simulink model "P2PHVDCMMC"  (R2024a)
settings: Solver=FixedStepDiscrete  StartTime=0.0  StopTime=10  RelTol=1e-3
PreLoadFcn:
  | % HVDCMMCInterconnectionParam
StartFcn:
  | tic
StopFcn:
  | toc
values from neighbouring files (symbols this model uses):
  C_PM = 1.758e-3    (= 0.001758)    [P2PHVDCMMCcode.m]
  Cg = 50e-9    (= 5e-08)    [P2PHVDCMMCcode.m]
  Fc = Fnom*3.37    (= 168.5)    [P2PHVDCMMCcode.m]
  Fnom = 50    [P2PHVDCMMCcode.m]
  HRM = 1    [P2PHVDCMMCcode.m]
  Ki_Ireg = 6    [P2PHVDCMMCcode.m]
  Ki_Preg = 1.0    (= 1)    [P2PHVDCMMCcode.m]
  Ki_Qreg = 1.0    (= 1)    [P2PHVDCMMCcode.m]
  Ki_VDCreg = 100    [P2PHVDCMMCcode.m]
  Kp_Ireg = 0.6    [P2PHVDCMMCcode.m]
  Kp_Preg = 0.5/3    (= 0.166666666667)    [P2PHVDCMMCcode.m]
  Kp_Qreg = 0.5/3    (= 0.166666666667)    [P2PHVDCMMCcode.m]
  Kp_VDCreg = 4    [P2PHVDCMMCcode.m]
  L_cable = 15e-3    (= 0.015)    [P2PHVDCMMCcode.m]
  Larm = Larm_pu*(Zb_ac/(2*pi*Fnom))    [P2PHVDCMMCcode.m]
  Larm_pu = 0.15    [P2PHVDCMMCcode.m]
  Lff = Larm_pu/2    (= 0.075)    [P2PHVDCMMCcode.m]
  Limits_Ireg = [ 2.0  -2.0]    [P2PHVDCMMCcode.m]
  Limits_Preg = [ 1.2, 0.8 ]    [P2PHVDCMMCcode.m]
  Limits_Qreg = [ 0.25, -0.25 ]    [P2PHVDCMMCcode.m]
  Limits_VDCreg = [ 2.0  -2.0]    [P2PHVDCMMCcode.m]
  Lxfo = 0.12    [P2PHVDCMMCcode.m]
  N = 6    [P2PHVDCMMCcode.m]
  Nb_PM = 36    [P2PHVDCMMCcode.m]
  Pnom = 1000e6    (= 1000000000)    [P2PHVDCMMCcode.m]
  R_cable = 0.5    [P2PHVDCMMCcode.m]
  R_startup = 400    [P2PHVDCMMCcode.m]
  Rarm = Rarm_pu*Zb_ac    [P2PHVDCMMCcode.m]
  Rff = Rarm_pu/2    (= 0.00075)    [P2PHVDCMMCcode.m]
  Rg = 100    [P2PHVDCMMCcode.m]
  Rxfo = 0.003    [P2PHVDCMMCcode.m]
  Slope_Qref = 0.5    [P2PHVDCMMCcode.m]
  Slope_Vdc_ref = Vnom_dc/5    (= 128000)    [P2PHVDCMMCcode.m]
  Tfault = 9999    [P2PHVDCMMCcode.m]
  Ts = Ts_Control    (= 4e-05)    [P2PHVDCMMCcode.m]
  Ts_Control = 40e-6    (= 4e-05)    [P2PHVDCMMCcode.m]
  Ts_dqn = 2e-5    (= 2e-05)    [P2PHVDCMMCcode.m]
  Ts_Power = 20e-6    (= 2e-05)    [P2PHVDCMMCcode.m]
  Vnom_dc = 640e3    (= 640000)    [P2PHVDCMMCcode.m]
  Vnom_prim = 400e3    (= 400000)    [P2PHVDCMMCcode.m]
  Vnom_sec = 333e3    (= 333000)    [P2PHVDCMMCcode.m]
  Ws = 2*pi*50    (= 314.159265359)    [P2PHVDCMMCcode.m]
undefined symbols (not defined in the file or in its folder): DiscIntNeverNeededParam, Discrete, DQN_Lib, gcbh, Int_DQNc_Mat, Mult_DQNc_Mat, Pcc, S, sps, sps_rtmsupport, spsMeanValueVariableFrequencyModel, spsPLL3phModel, SY3
libraries: simulink x38, spsControlledVoltageSourceLib x30, spsVoltageMeasurementLib x21, spsIdealSwitchLib x21, powerlib_extras x12, spsSecondOrderFilterLib x12, spsCurrentMeasurementLib x12, spsdq0toabcLib x9, spsMeanLib x8, spsMeanVariableFrequencyLib x8, spsabctodq0Lib x8, spsThreePhaseSeriesRLCBranchLib x7
(part 6 of 13)

== system P2PHVDCMMC/MMC AVG_Rec/Circulating current suppression/PI regulator with anti-windup D ==
  note: Anti-windup mechanism: Method of conditionnal integration
      |
      | The integration is suspended if saturation occurs and the
      | control error is of the same sign as the control signal.
      |
      | [1] L.Rundqwist, "Anti-Reset Windup for PID Controllers," Ph.D. Thesis TRFT-1033,
      | Departement of Automatic Control, Lund Institute of Technology, Lund, Sweeden, 1991.
  Error : Inport  SampleTime=Ts
  Compare To Zero : simulink/Logic and Bit Operations/Compare To Zero  relop=>  OutDataTypeStr=uint8  ZeroCross=off
  Compare To Zero1 : simulink/Logic and Bit Operations/Compare To Zero  relop=<  OutDataTypeStr=uint8  ZeroCross=off
  Constant : Constant  Value=0
  Constant1 : Constant  Value=UpperLimit
  Constant3 : Constant  Value=LowerLimit
  Discrete-Time Integrator : DiscreteIntegrator  IntegratorMethod=Integration: Trapezoidal  InitialCondition=Init  SampleTime=Ts  LimitOutput=on  UpperSaturationLimit=UpperLimit  LowerSaturationLimit=LowerLimit  ShowStatePort=on  ICPrevOutput=DiscIntNeverNeededParam  ICPrevScaledInput=DiscIntNeverNeededParam
  Kp4 : Gain  Gain=Kp  SaturateOnIntegerOverflow=on  SampleTime=Ts  OutDataTypeStr=Inherit: Same as input  ParamDataTypeStr=Inherit: Same as input
  Kp5 : Gain  Gain=Ki  SaturateOnIntegerOverflow=on  SampleTime=Ts  OutDataTypeStr=Inherit: Same as input  ParamDataTypeStr=Inherit: Same as input
  Logical Operator : Logic  AllPortsSameDT=off  OutDataTypeStr=boolean
  Logical Operator1 : Logic  AllPortsSameDT=off  OutDataTypeStr=boolean
  Logical Operator2 : Logic  Operator=OR  AllPortsSameDT=off  OutDataTypeStr=boolean
  Relational Operator : RelationalOperator  OutDataTypeStr=boolean  InputSameDT=off
  Relational Operator1 : RelationalOperator  Operator=<=  OutDataTypeStr=boolean  InputSameDT=off
  Saturation2 : Saturate  UpperLimit=UpperLimit  LowerLimit=LowerLimit  SampleTime=Ts
  Sum1 : Sum  InputSameDT=on  SaturateOnIntegerOverflow=on  SampleTime=Ts  OutDataTypeStr=Inherit: Same as first input
  Sum6 : Sum  InputSameDT=on  SaturateOnIntegerOverflow=on  SampleTime=Ts  OutDataTypeStr=Inherit: Same as first input
  Switch : Switch  Criteria=u2 > Threshold  SaturateOnIntegerOverflow=off  InputSameDT=off
  Zero-Order Hold : ZeroOrderHold  SampleTime=Ts
  Out : Outport  SampleTime=Ts  InitialOutput=0
  wires:
  Constant/1 -> Switch/1
  Zero-Order Hold/1 -> Sum1/2, Sum6/1
  Discrete-Time Integrator/State -> Sum1/1
  Sum1/1 -> Relational Operator1/1, Relational Operator/1
  Logical Operator2/1 -> Switch/2
  Relational Operator/1 -> Logical Operator/1  "UpperLimit_is_Reached"
  Relational Operator1/1 -> Logical Operator1/1  "LowerLimit_Is_Reached"
  Constant1/1 -> Relational Operator/2
  Constant3/1 -> Relational Operator1/2
  Compare To Zero/1 -> Logical Operator/2  "Error_is_positive"
  Logical Operator/1 -> Logical Operator2/1
  Logical Operator1/1 -> Logical Operator2/2
  Compare To Zero1/1 -> Logical Operator1/2  "Error_is_negative"
  Error/1 -> Compare To Zero1/1, Compare To Zero/1, Kp4/1, Kp5/1
  Sum6/1 -> Saturation2/1
  Kp4/1 -> Zero-Order Hold/1
  Discrete-Time Integrator/1 -> Sum6/2
  Saturation2/1 -> Out/1
  Switch/1 -> Discrete-Time Integrator/1
  Kp5/1 -> Switch/3

== system P2PHVDCMMC/MMC AVG_Rec/Circulating current suppression/PI regulator with anti-windup D1 ==
  note: Anti-windup mechanism: Method of conditionnal integration
      |
      | The integration is suspended if saturation occurs and the
      | control error is of the same sign as the control signal.
      |
      | [1] L.Rundqwist, "Anti-Reset Windup for PID Controllers," Ph.D. Thesis TRFT-1033,
      | Departement of Automatic Control, Lund Institute of Technology, Lund, Sweeden, 1991.
  Error : Inport  SampleTime=Ts
  Compare To Zero : simulink/Logic and Bit Operations/Compare To Zero  relop=>  OutDataTypeStr=uint8  ZeroCross=off
  Compare To Zero1 : simulink/Logic and Bit Operations/Compare To Zero  relop=<  OutDataTypeStr=uint8  ZeroCross=off
  Constant : Constant  Value=0
  Constant1 : Constant  Value=UpperLimit
  Constant3 : Constant  Value=LowerLimit
  Discrete-Time Integrator : DiscreteIntegrator  IntegratorMethod=Integration: Trapezoidal  InitialCondition=Init  SampleTime=Ts  LimitOutput=on  UpperSaturationLimit=UpperLimit  LowerSaturationLimit=LowerLimit  ShowStatePort=on  ICPrevOutput=DiscIntNeverNeededParam  ICPrevScaledInput=DiscIntNeverNeededParam
  Kp4 : Gain  Gain=Kp  SaturateOnIntegerOverflow=on  SampleTime=Ts  OutDataTypeStr=Inherit: Same as input  ParamDataTypeStr=Inherit: Same as input
  Kp5 : Gain  Gain=Ki  SaturateOnIntegerOverflow=on  SampleTime=Ts  OutDataTypeStr=Inherit: Same as input  ParamDataTypeStr=Inherit: Same as input
  Logical Operator : Logic  AllPortsSameDT=off  OutDataTypeStr=boolean
  Logical Operator1 : Logic  AllPortsSameDT=off  OutDataTypeStr=boolean
  Logical Operator2 : Logic  Operator=OR  AllPortsSameDT=off  OutDataTypeStr=boolean
  Relational Operator : RelationalOperator  OutDataTypeStr=boolean  InputSameDT=off
  Relational Operator1 : RelationalOperator  Operator=<=  OutDataTypeStr=boolean  InputSameDT=off
  Saturation2 : Saturate  UpperLimit=UpperLimit  LowerLimit=LowerLimit  SampleTime=Ts
  Sum1 : Sum  InputSameDT=on  SaturateOnIntegerOverflow=on  SampleTime=Ts  OutDataTypeStr=Inherit: Same as first input
  Sum6 : Sum  InputSameDT=on  SaturateOnIntegerOverflow=on  SampleTime=Ts  OutDataTypeStr=Inherit: Same as first input
  Switch : Switch  Criteria=u2 > Threshold  SaturateOnIntegerOverflow=off  InputSameDT=off
  Zero-Order Hold : ZeroOrderHold  SampleTime=Ts
  Out : Outport  SampleTime=Ts  InitialOutput=0
  wires:
  Kp5/1 -> Switch/3
  Switch/1 -> Discrete-Time Integrator/1
  Saturation2/1 -> Out/1
  Discrete-Time Integrator/1 -> Sum6/2
  Kp4/1 -> Zero-Order Hold/1
  Sum6/1 -> Saturation2/1
  Error/1 -> Kp5/1, Kp4/1, Compare To Zero/1, Compare To Zero1/1
  Compare To Zero1/1 -> Logical Operator1/2  "Error_is_negative"
  Logical Operator1/1 -> Logical Operator2/2
  Logical Operator/1 -> Logical Operator2/1
  Compare To Zero/1 -> Logical Operator/2  "Error_is_positive"
  Constant3/1 -> Relational Operator1/2
  Constant1/1 -> Relational Operator/2
  Relational Operator1/1 -> Logical Operator1/1  "LowerLimit_Is_Reached"
  Relational Operator/1 -> Logical Operator/1  "UpperLimit_is_Reached"
  Logical Operator2/1 -> Switch/2
  Sum1/1 -> Relational Operator/1, Relational Operator1/1
  Discrete-Time Integrator/State -> Sum1/1
  Zero-Order Hold/1 -> Sum6/1, Sum1/2
  Constant/1 -> Switch/1

== system P2PHVDCMMC/MMC AVG_Rec/Subsystem1/Circulating current suppression1 ==
  I_arm : Inport
  wt : Inport  Port=2
  Complex to Real-Imag2 : ComplexToRealImag
  Constant1 : Constant  Value=0
  Constant2 : Constant  Value=0
  Constant4 : Constant  Value=0
  Demux : Demux  Outputs=2
  Gain : Gain  Gain=0*Larm_pu
  Gain1 : Gain  Gain=0*Larm_pu
  Gain2 : Gain  Gain=-2
  I->pu1 : Gain  Gain=0.5  SaturateOnIntegerOverflow=on  OutDataTypeStr=Inherit: Same as input  ParamDataTypeStr=Inherit: Same as input
  I->pu4 : Gain  Gain=sqrt(3)*Vnom_prim/sqrt(2)/Pnom  SaturateOnIntegerOverflow=on  OutDataTypeStr=Inherit: Same as input  ParamDataTypeStr=Inherit: Same as input
  Mux1 : Mux  Inputs=3
  Mux2 : Mux  Inputs=2
  PI regulator with anti-windup D : Subsystem  DialogController=POWERSYS.PowerSysDialog  mask(Discrete PI Controller){Kp=1, Ki=5, Par_Limits=Limits_Ireg, Init=0, Ts=Ts}
      mask prompts: Kp "Proportional gain (Kp):"; Ki "Integral gain (Ki):"; Par_Limits "Output limits: [ Upper   Lower ]"; Init "Output initial value:"; Ts "Sample time:"
      mask help: This block implements a discrete PI controller.
      mask init:
      | UpperLimit=Par_Limits(1);
      | LowerLimit=Par_Limits(2);
      | power_initmask();
      mask Help: This block is part of a subset of blocks in the Extras library that does not have documentation associated with it, other than the block mask description.
      mask Display: disp('PI');
  PI regulator with anti-windup D1 : Subsystem  DialogController=POWERSYS.PowerSysDialog  mask(Discrete PI Controller){Kp=1, Ki=5, Par_Limits=Limits_Ireg, Init=0, Ts=Ts}
      mask prompts: Kp "Proportional gain (Kp):"; Ki "Integral gain (Ki):"; Par_Limits "Output limits: [ Upper   Lower ]"; Init "Output initial value:"; Ts "Sample time:"
      mask help: This block implements a discrete PI controller.
      mask init:
      | UpperLimit=Par_Limits(1);
      | LowerLimit=Par_Limits(2);
      | power_initmask();
      mask Help: This block is part of a subset of blocks in the Extras library that does not have documentation associated with it, other than the block mask description.
      mask Display: disp('PI');
  Rate Transition1 : RateTransition  OutPortSampleTime=Ts_Control
  Saturation1 : Saturate  UpperLimit=2  LowerLimit=-2
  Scope1 : Scope
  Selector1 : Selector  NumberOfDimensions=2  InputPortWidth=3  IndexOptions=Index vector (dialog),Index vector (dialog)  Indices=2,3  OutputSizes=1,1
  Sum1 : Sum  Inputs=-+|
  Sum78 : Sum  Inputs=|++
  Sum83 : Sum  Inputs=-+|
  Sum85 : Sum  Inputs=|+-
  dq0 to abc : spsdq0toabcLib/dq0 to abc  Alignment=90 degrees behind phase A axis
  V_diffi : Outport  VectorParamsAs1DForOutWhenUnconnected=off
  wires:
  I_arm/1 -> Selector1/1
  Gain2/1 -> dq0 to abc/2
  wt/1 -> Gain2/1
  Demux/1 -> Gain/1, Sum85/2
  Gain1/1 -> Sum78/2
  Demux/2 -> Gain1/1, Sum83/1
  dq0 to abc/1 -> Saturation1/1
  Constant1/1 -> Sum83/2
  Sum83/1 -> PI regulator with anti-windup D1/1(Error)
  Sum85/1 -> PI regulator with anti-windup D/1(Error)
  Sum78/1 -> Mux1/1
  Gain/1 -> Sum1/1
  Mux1/1 -> dq0 to abc/1
  PI regulator with anti-windup D/1(Out) -> Sum78/1
  PI regulator with anti-windup D1/1(Out) -> Sum1/2
  Sum1/1 -> Mux1/2
  Constant4/1 -> Mux1/3
  Constant2/1 -> Sum85/1
  Saturation1/1 -> V_diffi/1
  Selector1/1 -> Complex to Real-Imag2/1
  Mux2/1 -> Rate Transition1/1
  Complex to Real-Imag2/2 -> Mux2/2
  Complex to Real-Imag2/1 -> Mux2/1
  Rate Transition1/1 -> I->pu1/1
  I->pu1/1 -> I->pu4/1
  I->pu4/1 -> Demux/1, Scope1/1

== system P2PHVDCMMC/MMC AVG_Rec/Subsystem1/Subsystem ==
  g : Inport
  CVS{1..6} (6 alike) : spsControlledVoltageSourceLib/Controlled Voltage Source  Initialize=off  Source_Type=AC  Amplitude=0  Phase=0  Frequency=0  Measurements=None
  Constant2 : Constant  Value=Vnom_dc/2  SampleTime=Ts_Power
  Ground1 : spsGroundLib/Ground  LConnTagsString=a
  Subsystem : Subsystem
      settings: PortSchema="{\"entries\":[{\"content\":{\"sides\":[{\"content\":{\"connectorIds\":[\"In1\"]},\"type\":\"ConnectorPlacement.EquallySpacedRectSide\",\"uuid\":\"a5cee0a7-b338-4dc7-83bc-48872831f323\"},{\"content\":{\"side\":\"RIGHT\"},\"type\":\"ConnectorPlacement.EquallySpacedRectSide\",\"uuid\":\"ca317b42-2c00-457f-a5f3-7770b49527a9\"},{\"content\":{\"connectorIds\":[\"LConn1\",\"LConn2\",\"LConn3\"],\"side\":\"TOP\"},\"type\":\"ConnectorPlacement.EquallySpacedRectSide\",\"uuid\":\"77de2851-5038-4e86-9464-a1f28ff8b83a\"},{\"content\":{\"connectorIds\":[\"RConn1\",\"RConn2\",\"RConn3\"],\"side\":\"BOTTOM\"},\"type\":\"ConnectorPlacement.EquallySpacedRectSide\",\"uuid\":\"3c356faa-cb69-49bf-bf76-45ac18baf20f\"}]},\"type\":\"ConnectorPlacement.EquallySpacedConnector\",\"uuid\":\"03d4a433-e9ae-4343-977e-c6031a8cb266\"}],\"packageUris\":[\"http://schema.mathworks.com/mf0/Connector/R2020b\"],\"version\":\"1.0\"}"
  Subsystem1 : Subsystem
      settings: PortSchema="{\"entries\":[{\"content\":{\"sides\":[{\"content\":{\"connectorIds\":[\"In1\"]},\"type\":\"ConnectorPlacement.EquallySpacedRectSide\",\"uuid\":\"a5cee0a7-b338-4dc7-83bc-48872831f323\"},{\"content\":{\"side\":\"RIGHT\"},\"type\":\"ConnectorPlacement.EquallySpacedRectSide\",\"uuid\":\"ca317b42-2c00-457f-a5f3-7770b49527a9\"},{\"content\":{\"connectorIds\":[\"LConn1\",\"LConn2\",\"LConn3\"],\"side\":\"TOP\"},\"type\":\"ConnectorPlacement.EquallySpacedRectSide\",\"uuid\":\"77de2851-5038-4e86-9464-a1f28ff8b83a\"},{\"content\":{\"connectorIds\":[\"RConn1\",\"RConn2\",\"RConn3\"],\"side\":\"BOTTOM\"},\"type\":\"ConnectorPlacement.EquallySpacedRectSide\",\"uuid\":\"3c356faa-cb69-49bf-bf76-45ac18baf20f\"}]},\"type\":\"ConnectorPlacement.EquallySpacedConnector\",\"uuid\":\"03d4a433-e9ae-4343-977e-c6031a8cb266\"}],\"packageUris\":[\"http://schema.mathworks.com/mf0/Connector/R2020b\"],\"version\":\"1.0\"}"
  Voltage Measurement1 : spsVoltageMeasurementLib/Voltage Measurement  PhasorSimulation=off  OutputType=Complex  PSBequivalent=0
  Voltage Measurement2 : spsVoltageMeasurementLib/Voltage Measurement  PhasorSimulation=off  OutputType=Complex  PSBequivalent=0
  Voltage Measurement3 : spsVoltageMeasurementLib/Voltage Measurement  PhasorSimulation=off  OutputType=Complex  PSBequivalent=0
  + : PMIOPort  Side=Left
  +1 : PMIOPort  Port=2  Side=Left
  +3 : PMIOPort  Port=3  Side=Left
  - : PMIOPort  Port=4  Side=Right
  -1 : PMIOPort  Port=5  Side=Right
  -2 : PMIOPort  Port=6  Side=Right
  tag scope: Vdc12=global, Vdc13=global, Vdc1=global
  wires:
  Voltage Measurement2/1 -> [Vdc1]
  Voltage Measurement1/1 -> [Vdc12]
  Voltage Measurement3/1 -> [Vdc13]
  Constant2/1 -> CVS4/1, CVS5/1, CVS6/1, CVS1/1, CVS2/1, CVS3/1
  g/1 -> Subsystem/1(g), Subsystem1/1(g)
  connections:
  CVS6/RConn1 -- CVS2/LConn1 -- CVS1/LConn1 -- CVS4/RConn1 -- CVS5/RConn1 -- Ground1/LConn1 -- CVS3/LConn1
  Voltage Measurement2/LConn1 -- Subsystem/LConn1 -- +/RConn1
  Voltage Measurement2/LConn2 -- -/RConn1 -- Subsystem1/RConn1
  Voltage Measurement1/LConn2 -- -1/RConn1 -- Subsystem1/RConn2
  Voltage Measurement3/LConn2 -- Subsystem1/RConn3 -- -2/RConn1
  +1/RConn1 -- Subsystem/LConn2 -- Voltage Measurement1/LConn1
  +3/RConn1 -- Subsystem/LConn3 -- Voltage Measurement3/LConn1
  Subsystem/RConn2 -- CVS2/RConn1
  CVS1/RConn1 -- Subsystem/RConn1
  Subsystem/RConn3 -- CVS3/RConn1
  Subsystem1/LConn1 -- CVS4/LConn1
  Subsystem1/LConn2 -- CVS5/LConn1
  Subsystem1/LConn3 -- CVS6/LConn1

== system P2PHVDCMMC/Subsystem4/ACinv/Circulating current suppression2 ==
  I_arm : Inport
  wt : Inport  Port=2
  Complex to Real-Imag2 : ComplexToRealImag
  Constant1 : Constant  Value=0
  Constant2 : Constant  Value=0
  Constant4 : Constant  Value=0
  Demux : Demux  Outputs=2
  Demux4 : Demux  Outputs=2
  Gain : Gain  Gain=0*Larm_pu
  Gain1 : Gain  Gain=0*Larm_pu
  Gain2 : Gain  Gain=-2
  Gain4 : Gain  Gain=[ [zeros(1,N+4)] ; [0, 0,1 ,zeros(1,N+1)];[zeros(1,N+4)]]
  I->pu1 : Gain  Gain=0.5  SaturateOnIntegerOverflow=on  OutDataTypeStr=Inherit: Same as input  ParamDataTypeStr=Inherit: Same as input
  I->pu4 : Gain  Gain=sqrt(3)*Vnom_prim/sqrt(2)/Pnom  SaturateOnIntegerOverflow=on  OutDataTypeStr=Inherit: Same as input  ParamDataTypeStr=Inherit: Same as input
  Mux1 : Mux  Inputs=3
  Mux2 : Mux  Inputs=2
  Mux3 : Mux  Inputs=2
  PI regulator with anti-windup D : Subsystem  DialogController=POWERSYS.PowerSysDialog  mask(Discrete PI Controller){Kp=1, Ki=5, Par_Limits=Limits_Ireg, Init=0, Ts=Ts}
      mask prompts: Kp "Proportional gain (Kp):"; Ki "Integral gain (Ki):"; Par_Limits "Output limits: [ Upper   Lower ]"; Init "Output initial value:"; Ts "Sample time:"
      mask help: This block implements a discrete PI controller.
      mask init:
      | UpperLimit=Par_Limits(1);
      | LowerLimit=Par_Limits(2);
      | power_initmask();
      mask Help: This block is part of a subset of blocks in the Extras library that does not have documentation associated with it, other than the block mask description.
      mask Display: disp('PI');
  PI regulator with anti-windup D1 : Subsystem  DialogController=POWERSYS.PowerSysDialog  mask(Discrete PI Controller){Kp=1, Ki=5, Par_Limits=Limits_Ireg, Init=0, Ts=Ts}
      mask prompts: Kp "Proportional gain (Kp):"; Ki "Integral gain (Ki):"; Par_Limits "Output limits: [ Upper   Lower ]"; Init "Output initial value:"; Ts "Sample time:"
      mask help: This block implements a discrete PI controller.
      mask init:
      | UpperLimit=Par_Limits(1);
      | LowerLimit=Par_Limits(2);
      | power_initmask();
      mask Help: This block is part of a subset of blocks in the Extras library that does not have documentation associated with it, other than the block mask description.
      mask Display: disp('PI');
  Rate Transition1 : RateTransition  OutPortSampleTime=Ts_Control
  Rate Transition2 : RateTransition  OutPortSampleTime=Ts_Power
  Rate Transition3 : RateTransition  OutPortSampleTime=Ts_Power
  Real-Imag to Complex : RealImagToComplex
  Saturation1 : Saturate  UpperLimit=2  LowerLimit=-2
  Saturation2 : Saturate  UpperLimit=2  LowerLimit=-2
  Scope1 : Scope  Commented=on
  Selector1 : Selector  NumberOfDimensions=2  InputPortWidth=3  IndexOptions=Index vector (dialog),Index vector (dialog)  Indices=2,3  OutputSizes=1,1
  Sum1 : Sum  Inputs=-+|
  Sum78 : Sum  Inputs=|++
  Sum83 : Sum  Inputs=-+|
  Sum85 : Sum  Inputs=|+-
  dq0 to abc : spsdq0toabcLib/dq0 to abc  Alignment=90 degrees behind phase A axis
  V_diffi : Outport  VectorParamsAs1DForOutWhenUnconnected=off
  -2Uref_dq0 : Outport  Port=2
  wires:
  Rate Transition3/1 -> -2Uref_dq0/1
  Rate Transition2/1 -> V_diffi/1
  Mux3/1 -> Saturation2/1
  Real-Imag to Complex/1 -> Gain4/1
  Demux4/2 -> Real-Imag to Complex/2
  Gain4/1 -> Rate Transition3/1
  Demux4/1 -> Real-Imag to Complex/1
  I->pu4/1 -> Scope1/1, Demux/1
  I->pu1/1 -> I->pu4/1
  Rate Transition1/1 -> I->pu1/1
  Complex to Real-Imag2/1 -> Mux2/1
  Complex to Real-Imag2/2 -> Mux2/2
  Mux2/1 -> Rate Transition1/1
  Selector1/1 -> Complex to Real-Imag2/1
  Saturation1/1 -> Rate Transition2/1
  Constant2/1 -> Sum85/1
  Constant4/1 -> Mux1/3
  Sum1/1 -> Mux3/2, Mux1/2
  PI regulator with anti-windup D1/1(Out) -> Sum1/2
  PI regulator with anti-windup D/1(Out) -> Sum78/1
  Mux1/1 -> dq0 to abc/1
  Gain/1 -> Sum1/1
  Sum78/1 -> Mux1/1, Mux3/1
  Sum85/1 -> PI regulator with anti-windup D/1(Error)
  Sum83/1 -> PI regulator with anti-windup D1/1(Error)
  Constant1/1 -> Sum83/2
  dq0 to abc/1 -> Saturation1/1
  Demux/2 -> Sum83/1, Gain1/1
  Gain1/1 -> Sum78/2
  Demux/1 -> Sum85/2, Gain/1
  wt/1 -> Gain2/1
  Gain2/1 -> dq0 to abc/2
  I_arm/1 -> Selector1/1
  Saturation2/1 -> Demux4/1

== system P2PHVDCMMC/Subsystem4/ACrec/Circulating current suppression2 ==
  I_arm : Inport
  wt : Inport  Port=2
  Complex to Real-Imag2 : ComplexToRealImag
  Constant1 : Constant  Value=0
  Constant2 : Constant  Value=0
  Constant4 : Constant  Value=0
  Demux : Demux  Outputs=2
  Demux4 : Demux  Outputs=2
  Gain : Gain  Gain=0*Larm_pu
  Gain1 : Gain  Gain=0*Larm_pu
  Gain2 : Gain  Gain=-2
  Gain3 : Gain  Gain=[ [zeros(1,N+4)] ; [0, 0,1 ,zeros(1,N+1)];[zeros(1,N+4)]]
  I->pu1 : Gain  Gain=0.5  SaturateOnIntegerOverflow=on  OutDataTypeStr=Inherit: Same as input  ParamDataTypeStr=Inherit: Same as input
  I->pu4 : Gain  Gain=sqrt(3)*Vnom_prim/sqrt(2)/Pnom  SaturateOnIntegerOverflow=on  OutDataTypeStr=Inherit: Same as input  ParamDataTypeStr=Inherit: Same as input
  Mux1 : Mux  Inputs=3
  Mux2 : Mux  Inputs=2
  Mux3 : Mux  Inputs=2
  PI regulator with anti-windup D : Subsystem  DialogController=POWERSYS.PowerSysDialog  mask(Discrete PI Controller){Kp=1, Ki=5, Par_Limits=Limits_Ireg, Init=0, Ts=Ts}
      mask prompts: Kp "Proportional gain (Kp):"; Ki "Integral gain (Ki):"; Par_Limits "Output limits: [ Upper   Lower ]"; Init "Output initial value:"; Ts "Sample time:"
      mask help: This block implements a discrete PI controller.
      mask init:
      | UpperLimit=Par_Limits(1);
      | LowerLimit=Par_Limits(2);
      | power_initmask();
      mask Help: This block is part of a subset of blocks in the Extras library that does not have documentation associated with it, other than the block mask description.
      mask Display: disp('PI');
  PI regulator with anti-windup D1 : Subsystem  DialogController=POWERSYS.PowerSysDialog  mask(Discrete PI Controller){Kp=1, Ki=5, Par_Limits=Limits_Ireg, Init=0, Ts=Ts}
      mask prompts: Kp "Proportional gain (Kp):"; Ki "Integral gain (Ki):"; Par_Limits "Output limits: [ Upper   Lower ]"; Init "Output initial value:"; Ts "Sample time:"
      mask help: This block implements a discrete PI controller.
      mask init:
      | UpperLimit=Par_Limits(1);
      | LowerLimit=Par_Limits(2);
      | power_initmask();
      mask Help: This block is part of a subset of blocks in the Extras library that does not have documentation associated with it, other than the block mask description.
      mask Display: disp('PI');
  Rate Transition1 : RateTransition  OutPortSampleTime=Ts_Control
  Rate Transition2 : RateTransition  OutPortSampleTime=Ts_Power
  Rate Transition3 : RateTransition  OutPortSampleTime=Ts_Power
  Real-Imag to Complex : RealImagToComplex
  Saturation1 : Saturate  UpperLimit=2  LowerLimit=-2
  Saturation2 : Saturate  UpperLimit=2  LowerLimit=-2
  Scope1 : Scope  Commented=on
  Selector1 : Selector  NumberOfDimensions=2  InputPortWidth=3  IndexOptions=Index vector (dialog),Index vector (dialog)  Indices=2,3  OutputSizes=1,1
  Sum1 : Sum  Inputs=-+|
  Sum78 : Sum  Inputs=|++
  Sum83 : Sum  Inputs=-+|
  Sum85 : Sum  Inputs=|+-
  dq0 to abc : spsdq0toabcLib/dq0 to abc  Alignment=90 degrees behind phase A axis
  V_diffi : Outport  VectorParamsAs1DForOutWhenUnconnected=off
  -2Uref_dq0 : Outport  Port=2
  wires:
  Saturation2/1 -> Demux4/1
  I_arm/1 -> Selector1/1
  Gain2/1 -> dq0 to abc/2
  wt/1 -> Gain2/1
  Demux/1 -> Gain/1, Sum85/2
  Gain1/1 -> Sum78/2
  Demux/2 -> Gain1/1, Sum83/1
  dq0 to abc/1 -> Saturation1/1
  Constant1/1 -> Sum83/2
  Sum83/1 -> PI regulator with anti-windup D1/1(Error)
  Sum85/1 -> PI regulator with anti-windup D/1(Error)
  Sum78/1 -> Mux3/1, Mux1/1
  Gain/1 -> Sum1/1
  Mux1/1 -> dq0 to abc/1
  PI regulator with anti-windup D/1(Out) -> Sum78/1
  PI regulator with anti-windup D1/1(Out) -> Sum1/2
  Sum1/1 -> Mux1/2, Mux3/2
  Constant4/1 -> Mux1/3
  Constant2/1 -> Sum85/1
  Saturation1/1 -> Rate Transition2/1
  Selector1/1 -> Complex to Real-Imag2/1
  Mux2/1 -> Rate Transition1/1
  Complex to Real-Imag2/2 -> Mux2/2
  Complex to Real-Imag2/1 -> Mux2/1
  Rate Transition1/1 -> I->pu1/1
  I->pu1/1 -> I->pu4/1
  I->pu4/1 -> Demux/1, Scope1/1
  Demux4/1 -> Real-Imag to Complex/1
  Gain3/1 -> Rate Transition3/1
  Demux4/2 -> Real-Imag to Complex/2
  Real-Imag to Complex/1 -> Gain3/1
  Mux3/1 -> Saturation2/1
  Rate Transition2/1 -> V_diffi/1
  Rate Transition3/1 -> -2Uref_dq0/1

== system P2PHVDCMMC/Control _DQn_inv/PLL, Measurements and Transformation1/PLL (3ph)/Model ==
  note: vq
  Vdq : Inport
  Automatic Gain Control : Subsystem  TreatAsAtomicUnit=on
  Constant1 : Constant  Value=sps.AGC  SampleTime=Ts
  Constant4 : Constant  Value=2*pi  SampleTime=Ts
  Discrete : Subsystem  DialogController=POWERSYS.PowerSysDialog  VariantControl=PID_Discrete  mask(Discrete PID Controller){Kp=sps.Kp, Ki=sps.Ki, Kd=sps.Kd, TcD=sps.TcD, Par_Limits=[inf 0], Init=2*pi*sps.Finit, Ts=Ts}
      mask prompts: Kp "Proportional gain (Kp):"; Ki "Integral gain (Ki):"; Kd "Derivative gain (Kd):"; TcD "Time constant for derivative filter (s):"; Par_Limits "Output limits: [ Upper   Lower ]"; Init "Output initial value:"; Ts "Sample time:"
      mask help: This block implements a discrete PID controller.
      mask Display: disp('PID');
  Discrete-Time Integrator : DiscreteIntegrator  ExternalReset=rising  InitialConditionSource=external  InitialCondition=sps.Phase_Init*pi/180  SampleTime=Ts  ShowStatePort=on  ICPrevOutput=DiscIntNeverNeededParam  ICPrevScaledInput=DiscIntNeverNeededParam
  Divide : Product
  Gain10 : Gain  Gain=1/2/pi  SaturateOnIntegerOverflow=on  OutDataTypeStr=Inherit: Same as input  ParamDataTypeStr=Inherit: Same as input
  Initial : InitialCondition  Value=sps.Phase_Init*pi/180
  Rate Limiter : RateLimiter  RisingSlewLimit=sps.MaxRateChangeFreq  FallingSlewLimit=-sps.MaxRateChangeFreq  SampleTimeMode=inherited  InitialCondition=sps.Finit
  Relational Operator : RelationalOperator  Operator=>  OutDataTypeStr=boolean  InputSameDT=off
  Second-Order Filter : spsSecondOrderFilterLib/Second-Order Filter  FilterType=Lowpass  Fo=sps.FilterCutOffFreq  Zeta=0.707  Ts=Ts  Initialize=on  Vac_Init=[0 0 sps.Finit]  Vdc_Init=sps.Finit  PlotResponse=off  FreqRange=[1 500 1]
      settings: LibrarySourceBlock=|
      | sps_lib/Control/Filters/Second-Order
      | Filter
  Selector : Selector  Commented=on  InputPortWidth=3  IndexOptions=Index vector (dialog)  Indices=2  OutputSizes=1
  Selector1 : Selector  InputPortWidth=2  IndexOptions=Index vector (dialog)  Indices=2  OutputSizes=1
  Subtract : Sum  Inputs=+-
  Unit Delay : UnitDelay  InitialCondition=sps.Finit  SampleTime=Ts  HasFrameUpgradeWarning=on
  Variable Frequency Mean value : Subsystem  AncestorBlock=|  DialogController=POWERSYS.PowerSysDialog  LoadFcn=sps_rtmsupport('LoadFcn', gcbh);  StartFcn=sps_rtmsupport('StartFcn', gcbh);  StopFcn=sps_rtmsupport('StopFcn', gcbh);  mask(Mean (Variable Frequency)){Finit=sps.Finit, Fmin=sps.Fmin, Vinit=0, Ts=Ts}
      | sps_lib/Sensors and Measurements/Mean
      | (Variable Frequency)
      mask prompts: Finit "Initial frequency (Hz):"; Fmin "Minimum frequency (Hz):"; Vinit "Initial input (DC component):"; Ts "Sample time:"
      mask help:
      | Compute the mean value of input 2 over a running window of one cycle of frequency signal given by input 1.
      |
      | For the first cycle of initial frequency, the output is held to the value specified in the Initial input (DC component) parameter.
      |
      | The Minimum frequency parameter is used to determine the buffer size of the Variable Time Delay block used under the mask of the block.
      mask init:
      | block=gcb;
      | [WantBlockChoice,Ts,sps] = powericon('MeanVariableFrequencyInit',block,Finit,Fmin,Vinit,Ts);
      | powericon('SetInternalModels','set',block,WantBlockChoice);
      settings: CopyFcn=sps_rtmsupport('CopyFcn', gcbh);  DeleteFcn=sps_rtmsupport('DeleteFcn', gcbh);  UndoDeleteFcn=sps_rtmsupport('UndoDeleteFcn', gcbh);  ModelCloseFcn=sps_rtmsupport('ModelCloseFcn', gcbh);  PreSaveFcn=sps_rtmsupport('PreSaveFcn', gcbh);  PostSaveFcn=sps_rtmsupport('PostSaveFcn', gcbh);  NameChangeFcn=sps_rtmsupport('NameChangeFcn', gcbh);  PreCopyFcn=sps_rtmsupport('PreCopyFcn', gcbh);  OpenFcn=sps_rtmsupport('OpenFcn', gcbh, []);  CloseFcn=sps_rtmsupport('CloseFcn', gcbh);  PreDeleteFcn=sps_rtmsupport('PreDeleteFcn', gcbh);
      settings: LibrarySourceBlock=|
      | sps_lib/Sensors and Measurements/Mean
      | (Variable Frequency)
      mask Help: helpview(psbhelp);
      mask Display:
      | port_label('input',1,'Freq')
      | port_label('input',2,'In')
      | plot(0,0, 1,1)
      | plot([0.8 1], [0.75 0.75])
      | plot([0.85 .95], [0.35 0.65],[0.85 .95], [0.65 0.35])
  abc to dq0 : spsabctodq0Lib/abc to dq0  Commented=on  Alignment=90 degrees behind phase A axis
  Freq : Outport  VectorParamsAs1DForOutWhenUnconnected=off
  wt : Outport  Port=2  VectorParamsAs1DForOutWhenUnconnected=off
  wires:
  Rate Limiter/1 -> Second-Order Filter/1
  Gain10/1 -> Rate Limiter/1
  Vdq/1 -> Automatic Gain Control/2(Vdq), Selector1/1
  Second-Order Filter/1 -> Unit Delay/1
  Unit Delay/1 -> Automatic Gain Control/1(Freq), Variable Frequency Mean value/1(Freq), Freq/1
  Discrete-Time Integrator/1 -> wt/1
  Constant4/1 -> Subtract/2, Relational Operator/2
  abc to dq0/1 -> Selector/1
  Discrete/1(Out) -> Gain10/1, Discrete-Time Integrator/1  "W"
  Variable Frequency Mean value/1(Mean) -> Divide/1
  Automatic Gain Control/1(Gain) -> Divide/2
  Divide/1 -> Discrete/1(Err)
  Constant1/1 -> Automatic Gain Control/Enable
  Relational Operator/1 -> Discrete-Time Integrator/2
  Discrete-Time Integrator/State -> Subtract/1, Relational Operator/1
  Subtract/1 -> Initial/1
  Initial/1 -> Discrete-Time Integrator/3
  Selector1/1 -> Variable Frequency Mean value/2(vq)

== system P2PHVDCMMC/Control _DQn_inv/PLL, Measurements and Transformation1/PLL (3ph)2/Model ==
  note: vq
  Vdq : Inport
  Automatic Gain Control : Subsystem  TreatAsAtomicUnit=on
  Constant1 : Constant  Value=sps.AGC  SampleTime=Ts
  Constant4 : Constant  Value=2*pi  SampleTime=Ts
  Discrete : Subsystem  DialogController=POWERSYS.PowerSysDialog  VariantControl=PID_Discrete  mask(Discrete PID Controller){Kp=sps.Kp, Ki=sps.Ki, Kd=sps.Kd, TcD=sps.TcD, Par_Limits=[inf 0], Init=2*pi*sps.Finit, Ts=Ts}
      mask prompts: Kp "Proportional gain (Kp):"; Ki "Integral gain (Ki):"; Kd "Derivative gain (Kd):"; TcD "Time constant for derivative filter (s):"; Par_Limits "Output limits: [ Upper   Lower ]"; Init "Output initial value:"; Ts "Sample time:"
      mask help: This block implements a discrete PID controller.
      mask Display: disp('PID');
  Discrete-Time Integrator : DiscreteIntegrator  ExternalReset=rising  InitialConditionSource=external  InitialCondition=sps.Phase_Init*pi/180  SampleTime=Ts  ShowStatePort=on  ICPrevOutput=DiscIntNeverNeededParam  ICPrevScaledInput=DiscIntNeverNeededParam
  Divide : Product
  Gain10 : Gain  Gain=1/2/pi  SaturateOnIntegerOverflow=on  OutDataTypeStr=Inherit: Same as input  ParamDataTypeStr=Inherit: Same as input
  Initial : InitialCondition  Value=sps.Phase_Init*pi/180
  MATLAB Function : MATLAB Function  TreatAsAtomicUnit=on
  Mux : Mux  Inputs=2
  Rate Limiter : RateLimiter  RisingSlewLimit=sps.MaxRateChangeFreq  FallingSlewLimit=-sps.MaxRateChangeFreq  SampleTimeMode=inherited  InitialCondition=sps.Finit
  Rate Transition3 : RateTransition  OutPortSampleTime=Ts_Control
  Relational Operator : RelationalOperator  Operator=>  OutDataTypeStr=boolean  InputSameDT=off
  Second-Order Filter : spsSecondOrderFilterLib/Second-Order Filter  FilterType=Lowpass  Fo=sps.FilterCutOffFreq  Zeta=0.707  Ts=Ts  Initialize=on  Vac_Init=[0 0 sps.Finit]  Vdc_Init=sps.Finit  PlotResponse=off  FreqRange=[1 500 1]
      settings: LibrarySourceBlock=|
      | sps_lib/Control/Filters/Second-Order
      | Filter
  Selector1 : Selector  InputPortWidth=2  IndexOptions=Index vector (dialog)  Indices=2  OutputSizes=1
  Subtract : Sum  Inputs=+-
  Sum : Sum  Inputs=|+-
  Unit Delay : UnitDelay  InitialCondition=sps.Finit  SampleTime=Ts  HasFrameUpgradeWarning=on
  Variable Frequency Mean value : Subsystem  AncestorBlock=|  DialogController=POWERSYS.PowerSysDialog  LoadFcn=sps_rtmsupport('LoadFcn', gcbh);  StartFcn=sps_rtmsupport('StartFcn', gcbh);  StopFcn=sps_rtmsupport('StopFcn', gcbh);  mask(Mean (Variable Frequency)){Finit=sps.Finit, Fmin=sps.Fmin, Vinit=0, Ts=Ts}
      | sps_lib/Sensors and Measurements/Mean
      | (Variable Frequency)
      mask prompts: Finit "Initial frequency (Hz):"; Fmin "Minimum frequency (Hz):"; Vinit "Initial input (DC component):"; Ts "Sample time:"
      mask help:
      | Compute the mean value of input 2 over a running window of one cycle of frequency signal given by input 1.
      |
      | For the first cycle of initial frequency, the output is held to the value specified in the Initial input (DC component) parameter.
      |
      | The Minimum frequency parameter is used to determine the buffer size of the Variable Time Delay block used under the mask of the block.
      mask init:
      | block=gcb;
      | [WantBlockChoice,Ts,sps] = powericon('MeanVariableFrequencyInit',block,Finit,Fmin,Vinit,Ts);
      | powericon('SetInternalModels','set',block,WantBlockChoice);
      settings: CopyFcn=sps_rtmsupport('CopyFcn', gcbh);  DeleteFcn=sps_rtmsupport('DeleteFcn', gcbh);  UndoDeleteFcn=sps_rtmsupport('UndoDeleteFcn', gcbh);  ModelCloseFcn=sps_rtmsupport('ModelCloseFcn', gcbh);  PreSaveFcn=sps_rtmsupport('PreSaveFcn', gcbh);  PostSaveFcn=sps_rtmsupport('PostSaveFcn', gcbh);  NameChangeFcn=sps_rtmsupport('NameChangeFcn', gcbh);  PreCopyFcn=sps_rtmsupport('PreCopyFcn', gcbh);  OpenFcn=sps_rtmsupport('OpenFcn', gcbh, []);  CloseFcn=sps_rtmsupport('CloseFcn', gcbh);  PreDeleteFcn=sps_rtmsupport('PreDeleteFcn', gcbh);
      settings: LibrarySourceBlock=|
      | sps_lib/Sensors and Measurements/Mean
      | (Variable Frequency)
      mask Help: helpview(psbhelp);
      mask Display:
      | port_label('input',1,'Freq')
      | port_label('input',2,'In')
      | plot(0,0, 1,1)
      | plot([0.8 1], [0.75 0.75])
      | plot([0.85 .95], [0.35 0.65],[0.85 .95], [0.65 0.35])
  Freq : Outport  VectorParamsAs1DForOutWhenUnconnected=off
  wt : Outport  Port=2  VectorParamsAs1DForOutWhenUnconnected=off
  wires:
  Rate Limiter/1 -> Second-Order Filter/1
  Gain10/1 -> Rate Limiter/1
  Second-Order Filter/1 -> Unit Delay/1
  Unit Delay/1 -> Automatic Gain Control/1(Freq), Variable Frequency Mean value/1(Freq), Freq/1
  Constant4/1 -> Subtract/2, Relational Operator/2
  Discrete/1(Out) -> Gain10/1, Discrete-Time Integrator/1  "W"
  Variable Frequency Mean value/1(Mean) -> Divide/1
  Automatic Gain Control/1(Gain) -> Divide/2
  Divide/1 -> Discrete/1(Err)
  Constant1/1 -> Automatic Gain Control/Enable
  Relational Operator/1 -> Discrete-Time Integrator/2
  Discrete-Time Integrator/State -> Subtract/1, Relational Operator/1
  Subtract/1 -> Initial/1
  Initial/1 -> Discrete-Time Integrator/3
  Selector1/1 -> Variable Frequency Mean value/2(vq)
  Sum/1 -> MATLAB Function/2(wt)
  Discrete-Time Integrator/1 -> Sum/1, wt/1
  MATLAB Function/1(d) -> Mux/1
  MATLAB Function/2(q) -> Mux/2
  Mux/1 -> Automatic Gain Control/2(Vdq), Selector1/1
  Vdq/1 -> MATLAB Function/1(DQ)
  [wt0] -> Rate Transition3/1
  Rate Transition3/1 -> Sum/2

== system P2PHVDCMMC/Control _DQn_rec/PLL, Measurements and Transformation1/PLL (3ph)/Model ==
  note: vq
  Vdq : Inport
  Automatic Gain Control : Subsystem  TreatAsAtomicUnit=on
  Constant1 : Constant  Value=sps.AGC  SampleTime=Ts
  Constant4 : Constant  Value=2*pi  SampleTime=Ts
  Discrete : Subsystem  DialogController=POWERSYS.PowerSysDialog  VariantControl=PID_Discrete  mask(Discrete PID Controller){Kp=sps.Kp, Ki=sps.Ki, Kd=sps.Kd, TcD=sps.TcD, Par_Limits=[inf 0], Init=2*pi*sps.Finit, Ts=Ts}
      mask prompts: Kp "Proportional gain (Kp):"; Ki "Integral gain (Ki):"; Kd "Derivative gain (Kd):"; TcD "Time constant for derivative filter (s):"; Par_Limits "Output limits: [ Upper   Lower ]"; Init "Output initial value:"; Ts "Sample time:"
      mask help: This block implements a discrete PID controller.
      mask Display: disp('PID');
  Discrete-Time Integrator : DiscreteIntegrator  ExternalReset=rising  InitialConditionSource=external  InitialCondition=sps.Phase_Init*pi/180  SampleTime=Ts  ShowStatePort=on  ICPrevOutput=DiscIntNeverNeededParam  ICPrevScaledInput=DiscIntNeverNeededParam
  Divide : Product
  Gain10 : Gain  Gain=1/2/pi  SaturateOnIntegerOverflow=on  OutDataTypeStr=Inherit: Same as input  ParamDataTypeStr=Inherit: Same as input
  Initial : InitialCondition  Value=sps.Phase_Init*pi/180
  Rate Limiter : RateLimiter  RisingSlewLimit=sps.MaxRateChangeFreq  FallingSlewLimit=-sps.MaxRateChangeFreq  SampleTimeMode=inherited  InitialCondition=sps.Finit
  Relational Operator : RelationalOperator  Operator=>  OutDataTypeStr=boolean  InputSameDT=off
  Second-Order Filter : spsSecondOrderFilterLib/Second-Order Filter  FilterType=Lowpass  Fo=sps.FilterCutOffFreq  Zeta=0.707  Ts=Ts  Initialize=on  Vac_Init=[0 0 sps.Finit]  Vdc_Init=sps.Finit  PlotResponse=off  FreqRange=[1 500 1]
      settings: LibrarySourceBlock=|
      | sps_lib/Control/Filters/Second-Order
      | Filter
  Selector : Selector  Commented=on  InputPortWidth=3  IndexOptions=Index vector (dialog)  Indices=2  OutputSizes=1
  Selector1 : Selector  InputPortWidth=2  IndexOptions=Index vector (dialog)  Indices=2  OutputSizes=1
  Subtract : Sum  Inputs=+-
  Unit Delay : UnitDelay  InitialCondition=sps.Finit  SampleTime=Ts  HasFrameUpgradeWarning=on
  Variable Frequency Mean value : Subsystem  AncestorBlock=|  DialogController=POWERSYS.PowerSysDialog  LoadFcn=sps_rtmsupport('LoadFcn', gcbh);  StartFcn=sps_rtmsupport('StartFcn', gcbh);  StopFcn=sps_rtmsupport('StopFcn', gcbh);  mask(Mean (Variable Frequency)){Finit=sps.Finit, Fmin=sps.Fmin, Vinit=0, Ts=Ts}
      | sps_lib/Sensors and Measurements/Mean
      | (Variable Frequency)
      mask prompts: Finit "Initial frequency (Hz):"; Fmin "Minimum frequency (Hz):"; Vinit "Initial input (DC component):"; Ts "Sample time:"
      mask help:
      | Compute the mean value of input 2 over a running window of one cycle of frequency signal given by input 1.
      |
      | For the first cycle of initial frequency, the output is held to the value specified in the Initial input (DC component) parameter.
      |
      | The Minimum frequency parameter is used to determine the buffer size of the Variable Time Delay block used under the mask of the block.
      mask init:
      | block=gcb;
      | [WantBlockChoice,Ts,sps] = powericon('MeanVariableFrequencyInit',block,Finit,Fmin,Vinit,Ts);
      | powericon('SetInternalModels','set',block,WantBlockChoice);
      settings: CopyFcn=sps_rtmsupport('CopyFcn', gcbh);  DeleteFcn=sps_rtmsupport('DeleteFcn', gcbh);  UndoDeleteFcn=sps_rtmsupport('UndoDeleteFcn', gcbh);  ModelCloseFcn=sps_rtmsupport('ModelCloseFcn', gcbh);  PreSaveFcn=sps_rtmsupport('PreSaveFcn', gcbh);  PostSaveFcn=sps_rtmsupport('PostSaveFcn', gcbh);  NameChangeFcn=sps_rtmsupport('NameChangeFcn', gcbh);  PreCopyFcn=sps_rtmsupport('PreCopyFcn', gcbh);  OpenFcn=sps_rtmsupport('OpenFcn', gcbh, []);  CloseFcn=sps_rtmsupport('CloseFcn', gcbh);  PreDeleteFcn=sps_rtmsupport('PreDeleteFcn', gcbh);
      settings: LibrarySourceBlock=|
      | sps_lib/Sensors and Measurements/Mean
      | (Variable Frequency)
      mask Help: helpview(psbhelp);
      mask Display:
      | port_label('input',1,'Freq')
      | port_label('input',2,'In')
      | plot(0,0, 1,1)
      | plot([0.8 1], [0.75 0.75])
      | plot([0.85 .95], [0.35 0.65],[0.85 .95], [0.65 0.35])
  abc to dq0 : spsabctodq0Lib/abc to dq0  Commented=on  Alignment=90 degrees behind phase A axis
  Freq : Outport  VectorParamsAs1DForOutWhenUnconnected=off
  wt : Outport  Port=2  VectorParamsAs1DForOutWhenUnconnected=off
  wires:
  Rate Limiter/1 -> Second-Order Filter/1
  Gain10/1 -> Rate Limiter/1
  Vdq/1 -> Automatic Gain Control/2(Vdq), Selector1/1
  Second-Order Filter/1 -> Unit Delay/1
  Unit Delay/1 -> Automatic Gain Control/1(Freq), Variable Frequency Mean value/1(Freq), Freq/1
  Discrete-Time Integrator/1 -> wt/1
  Constant4/1 -> Subtract/2, Relational Operator/2
  abc to dq0/1 -> Selector/1
  Discrete/1(Out) -> Gain10/1, Discrete-Time Integrator/1  "W"
  Variable Frequency Mean value/1(Mean) -> Divide/1
  Automatic Gain Control/1(Gain) -> Divide/2
  Divide/1 -> Discrete/1(Err)
  Constant1/1 -> Automatic Gain Control/Enable
  Relational Operator/1 -> Discrete-Time Integrator/2
  Discrete-Time Integrator/State -> Subtract/1, Relational Operator/1
  Subtract/1 -> Initial/1
  Initial/1 -> Discrete-Time Integrator/3
  Selector1/1 -> Variable Frequency Mean value/2(vq)

== system P2PHVDCMMC/Control _DQn_rec/PLL, Measurements and Transformation1/PLL (3ph)2/Model ==
  note: vq
  Vdq : Inport
  Automatic Gain Control : Subsystem  TreatAsAtomicUnit=on
  Constant1 : Constant  Value=sps.AGC  SampleTime=Ts
  Constant4 : Constant  Value=2*pi  SampleTime=Ts
  Discrete : Subsystem  DialogController=POWERSYS.PowerSysDialog  VariantControl=PID_Discrete  mask(Discrete PID Controller){Kp=sps.Kp, Ki=sps.Ki, Kd=sps.Kd, TcD=sps.TcD, Par_Limits=[inf 0], Init=2*pi*sps.Finit, Ts=Ts}
      mask prompts: Kp "Proportional gain (Kp):"; Ki "Integral gain (Ki):"; Kd "Derivative gain (Kd):"; TcD "Time constant for derivative filter (s):"; Par_Limits "Output limits: [ Upper   Lower ]"; Init "Output initial value:"; Ts "Sample time:"
      mask help: This block implements a discrete PID controller.
      mask Display: disp('PID');
  Discrete-Time Integrator : DiscreteIntegrator  ExternalReset=rising  InitialConditionSource=external  InitialCondition=sps.Phase_Init*pi/180  SampleTime=Ts  ShowStatePort=on  ICPrevOutput=DiscIntNeverNeededParam  ICPrevScaledInput=DiscIntNeverNeededParam
  Divide : Product
  Gain10 : Gain  Gain=1/2/pi  SaturateOnIntegerOverflow=on  OutDataTypeStr=Inherit: Same as input  ParamDataTypeStr=Inherit: Same as input
  Initial : InitialCondition  Value=sps.Phase_Init*pi/180
  MATLAB Function : MATLAB Function  TreatAsAtomicUnit=on
  Mux : Mux  Inputs=2
  Rate Limiter : RateLimiter  RisingSlewLimit=sps.MaxRateChangeFreq  FallingSlewLimit=-sps.MaxRateChangeFreq  SampleTimeMode=inherited  InitialCondition=sps.Finit
  Rate Transition3 : RateTransition  OutPortSampleTime=Ts_Control
  Relational Operator : RelationalOperator  Operator=>  OutDataTypeStr=boolean  InputSameDT=off
  Second-Order Filter : spsSecondOrderFilterLib/Second-Order Filter  FilterType=Lowpass  Fo=sps.FilterCutOffFreq  Zeta=0.707  Ts=Ts  Initialize=on  Vac_Init=[0 0 sps.Finit]  Vdc_Init=sps.Finit  PlotResponse=off  FreqRange=[1 500 1]
      settings: LibrarySourceBlock=|
      | sps_lib/Control/Filters/Second-Order
      | Filter
  Selector1 : Selector  InputPortWidth=2  IndexOptions=Index vector (dialog)  Indices=2  OutputSizes=1
  Subtract : Sum  Inputs=+-
  Sum : Sum  Inputs=|+-
  Unit Delay : UnitDelay  InitialCondition=sps.Finit  SampleTime=Ts  HasFrameUpgradeWarning=on
  Variable Frequency Mean value : Subsystem  AncestorBlock=|  DialogController=POWERSYS.PowerSysDialog  LoadFcn=sps_rtmsupport('LoadFcn', gcbh);  StartFcn=sps_rtmsupport('StartFcn', gcbh);  StopFcn=sps_rtmsupport('StopFcn', gcbh);  mask(Mean (Variable Frequency)){Finit=sps.Finit, Fmin=sps.Fmin, Vinit=0, Ts=Ts}
      | sps_lib/Sensors and Measurements/Mean
      | (Variable Frequency)
      mask prompts: Finit "Initial frequency (Hz):"; Fmin "Minimum frequency (Hz):"; Vinit "Initial input (DC component):"; Ts "Sample time:"
      mask help:
      | Compute the mean value of input 2 over a running window of one cycle of frequency signal given by input 1.
      |
      | For the first cycle of initial frequency, the output is held to the value specified in the Initial input (DC component) parameter.
      |
      | The Minimum frequency parameter is used to determine the buffer size of the Variable Time Delay block used under the mask of the block.
      mask init:
      | block=gcb;
      | [WantBlockChoice,Ts,sps] = powericon('MeanVariableFrequencyInit',block,Finit,Fmin,Vinit,Ts);
      | powericon('SetInternalModels','set',block,WantBlockChoice);
      settings: CopyFcn=sps_rtmsupport('CopyFcn', gcbh);  DeleteFcn=sps_rtmsupport('DeleteFcn', gcbh);  UndoDeleteFcn=sps_rtmsupport('UndoDeleteFcn', gcbh);  ModelCloseFcn=sps_rtmsupport('ModelCloseFcn', gcbh);  PreSaveFcn=sps_rtmsupport('PreSaveFcn', gcbh);  PostSaveFcn=sps_rtmsupport('PostSaveFcn', gcbh);  NameChangeFcn=sps_rtmsupport('NameChangeFcn', gcbh);  PreCopyFcn=sps_rtmsupport('PreCopyFcn', gcbh);  OpenFcn=sps_rtmsupport('OpenFcn', gcbh, []);  CloseFcn=sps_rtmsupport('CloseFcn', gcbh);  PreDeleteFcn=sps_rtmsupport('PreDeleteFcn', gcbh);
      settings: LibrarySourceBlock=|
      | sps_lib/Sensors and Measurements/Mean
      | (Variable Frequency)
      mask Help: helpview(psbhelp);
      mask Display:
      | port_label('input',1,'Freq')
      | port_label('input',2,'In')
      | plot(0,0, 1,1)
      | plot([0.8 1], [0.75 0.75])
      | plot([0.85 .95], [0.35 0.65],[0.85 .95], [0.65 0.35])
  Freq : Outport  VectorParamsAs1DForOutWhenUnconnected=off
  wt : Outport  Port=2  VectorParamsAs1DForOutWhenUnconnected=off
  wires:
  Rate Limiter/1 -> Second-Order Filter/1
  Gain10/1 -> Rate Limiter/1
  Second-Order Filter/1 -> Unit Delay/1
  Unit Delay/1 -> Automatic Gain Control/1(Freq), Variable Frequency Mean value/1(Freq), Freq/1
  Constant4/1 -> Subtract/2, Relational Operator/2
  Discrete/1(Out) -> Gain10/1, Discrete-Time Integrator/1  "W"
  Variable Frequency Mean value/1(Mean) -> Divide/1
  Automatic Gain Control/1(Gain) -> Divide/2
  Divide/1 -> Discrete/1(Err)
  Constant1/1 -> Automatic Gain Control/Enable
  Relational Operator/1 -> Discrete-Time Integrator/2
  Discrete-Time Integrator/State -> Subtract/1, Relational Operator/1
  Subtract/1 -> Initial/1
  Initial/1 -> Discrete-Time Integrator/3
  Selector1/1 -> Variable Frequency Mean value/2(vq)
  Sum/1 -> MATLAB Function/2(wt)
  Discrete-Time Integrator/1 -> Sum/1, wt/1
  MATLAB Function/1(d) -> Mux/1
  MATLAB Function/2(q) -> Mux/2
  Mux/1 -> Automatic Gain Control/2(Vdq), Selector1/1
  Vdq/1 -> MATLAB Function/1(DQ)
  [wt0] -> Rate Transition3/1
  Rate Transition3/1 -> Sum/2

== system P2PHVDCMMC/MMC AVG_Inv/Subsystem3/Subsystem/Subsystem ==
  g : Inport
  cb1 : spsIdealSwitchLib/Ideal Switch  Ron=0.001  Lon=0  IC=0  Rs=1e6  Cs=inf  Measurements=off
  cb2 : spsIdealSwitchLib/Ideal Switch  Ron=0.001  Lon=0  IC=0  Rs=1e6  Cs=inf  Measurements=off
  cb3 : spsIdealSwitchLib/Ideal Switch  Ron=0.001  Lon=0  IC=0  Rs=1e6  Cs=inf  Measurements=off
  1 : PMIOPort  Side=Left
  2 : PMIOPort  Port=2  Side=Left
  3 : PMIOPort  Port=3  Side=Left
  4 : PMIOPort  Port=4  Side=Right
  5 : PMIOPort  Port=5  Side=Right
  6 : PMIOPort  Port=6  Side=Right
  wires:
  g/1 -> cb3/1, cb2/1, cb1/1
  connections:
  cb3/RConn1 -- 6/RConn1
  cb3/LConn1 -- 3/RConn1
  cb2/RConn1 -- 5/RConn1
  cb1/LConn1 -- 1/RConn1
  cb1/RConn1 -- 4/RConn1
  cb2/LConn1 -- 2/RConn1

== system P2PHVDCMMC/MMC AVG_Inv/Subsystem3/Subsystem/Subsystem1 ==
  g : Inport
  cb4 : spsIdealSwitchLib/Ideal Switch  Ron=0.001  Lon=0  IC=0  Rs=1e6  Cs=inf  Measurements=off
  cb5 : spsIdealSwitchLib/Ideal Switch  Ron=0.001  Lon=0  IC=0  Rs=1e6  Cs=inf  Measurements=off
  cb6 : spsIdealSwitchLib/Ideal Switch  Ron=0.001  Lon=0  IC=0  Rs=1e6  Cs=inf  Measurements=off
  1 : PMIOPort  Side=Left
  2 : PMIOPort  Port=2  Side=Left
  3 : PMIOPort  Port=3  Side=Left
  4 : PMIOPort  Port=4  Side=Right
  5 : PMIOPort  Port=5  Side=Right
  6 : PMIOPort  Port=6  Side=Right
  wires:
  g/1 -> cb6/1, cb5/1, cb4/1
  connections:
  cb6/RConn1 -- 6/RConn1
  cb6/LConn1 -- 3/RConn1
  cb5/RConn1 -- 5/RConn1
  cb4/LConn1 -- 1/RConn1
  cb4/RConn1 -- 4/RConn1
  cb5/LConn1 -- 2/RConn1
